simulink model "MovimientoMotores"  (R2023b)
settings: Solver=VariableStepAuto  StartTime=0.0  StopTime=Inf  RelTol=1e-3
libraries: arduinolib x4
settings Model: Creator=Andrés  LastModifiedBy=Andrés

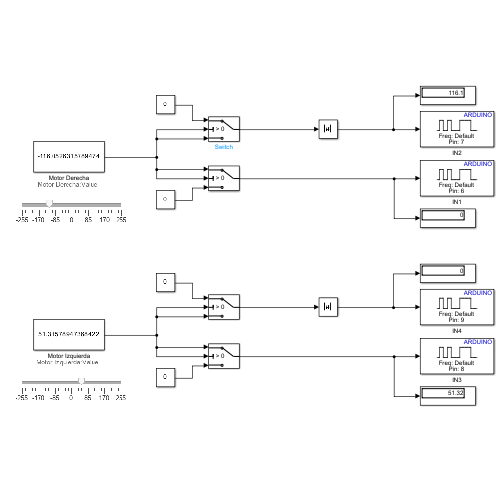
[thumbnail: Simulink's stored preview of the top-level diagram]
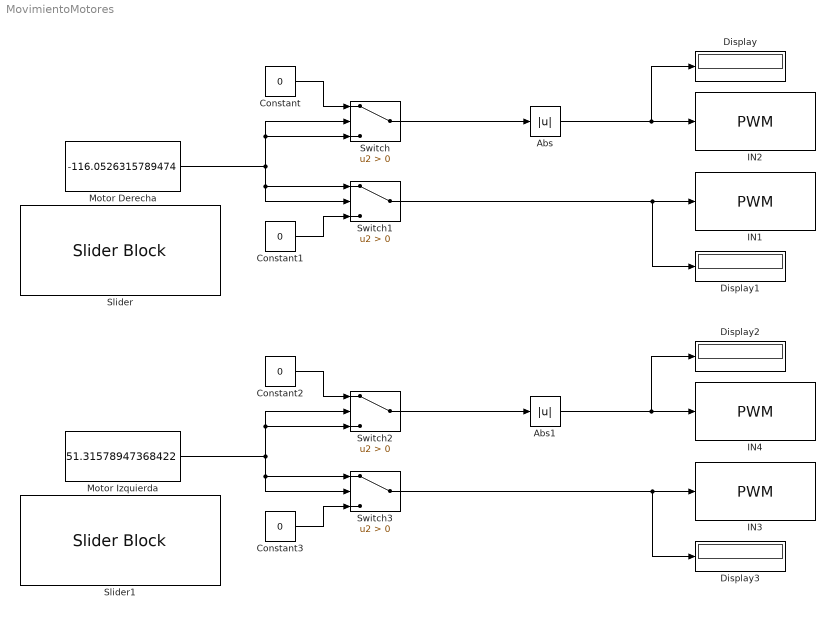
== system MovimientoMotores ==
  Abs : Abs  SaturateOnIntegerOverflow=off
  Abs1 : Abs  SaturateOnIntegerOverflow=off
  Constant{,1..3} (4 alike) : Constant  Value=0
  Display{,1..3} (4 alike) : Display
  IN1 : arduinolib/PWM  pinNumber=6  frequencyType=Default  desiredFrequency=490.2  achievableFrequency=490.2
  IN2 : arduinolib/PWM  pinNumber=7  frequencyType=Default  desiredFrequency=490.2  achievableFrequency=490.2
  IN3 : arduinolib/PWM  pinNumber=8  frequencyType=Default  desiredFrequency=490.2  achievableFrequency=490.2
  IN4 : arduinolib/PWM  pinNumber=9  frequencyType=Default  desiredFrequency=490.2  achievableFrequency=490.2
  Motor Derecha : Constant  Value=-116.0526315789474
  Motor Izquierda : Constant  Value=51.31578947368422
  Slider : SliderBlock  ScaleMin=-255  ScaleMax=255
  Slider1 : SliderBlock  ScaleMin=-255  ScaleMax=255
  Switch{,1..3} (4 alike) : Switch  Criteria=u2 > Threshold  SaturateOnIntegerOverflow=off  InputSameDT=off
  wires:
  Constant/1 -> Switch/1
  Switch1/1 -> Display1/1, IN1/1
  Switch/1 -> Abs/1
  Constant1/1 -> Switch1/3
  Motor Derecha/1 -> Switch/2, Switch/3, Switch1/2, Switch1/1
  Abs/1 -> Display/1, IN2/1
  Abs1/1 -> Display2/1, IN4/1
  Constant3/1 -> Switch3/3
  Switch2/1 -> Abs1/1
  Constant2/1 -> Switch2/1
  Switch3/1 -> Display3/1, IN3/1
  Motor Izquierda/1 -> Switch2/2, Switch2/3, Switch3/2, Switch3/1
